simulink model "controlador_PID"  (R2020a)
settings: Solver=VariableStepAuto  StartTime=0.0  StopTime=10.0  RelTol=1e-3
model workspace: external: MATLAB File D:\Ferran\Facultad\UNCuyo\Meca\Automática y Máquinas Eléctricas\Proyecto final\matlab2\parametros_y_especs\parametros_y_especif.m (data not in the file)
undefined symbols (not defined in the file): Ba, Ksa, Ksia
settings Model: Creator=Ferran  LastModifiedBy=Ferran

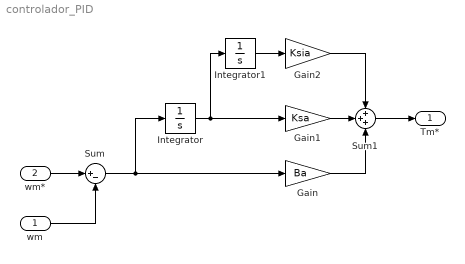
== system controlador_PID ==
  wm : Inport
  wm* : Inport  Port=2
  Gain : Gain  Gain=Ba
  Gain1 : Gain  Gain=Ksa
  Gain2 : Gain  Gain=Ksia
  Integrator : Integrator
  Integrator1 : Integrator
  Sum : Sum  Inputs=|+-
  Sum1 : Sum  Inputs=+++
  Tm* : Outport
  wires:
  wm*/1 -> Sum/1
  wm/1 -> Sum/2
  Sum/1 -> Gain/1, Integrator/1
  Integrator/1 -> Integrator1/1, Gain1/1
  Integrator1/1 -> Gain2/1
  Gain2/1 -> Sum1/1
  Gain1/1 -> Sum1/2
  Gain/1 -> Sum1/3
  Sum1/1 -> Tm*/1
